simulink model "TCS_SlipModelControl"  (R2023b)
settings: Solver=VariableStepAuto  StartTime=0.0  StopTime=10.0  RelTol=1e-3
libraries: autolibim x1
settings Model: Creator=ibaad  LastModifiedBy=ibaad

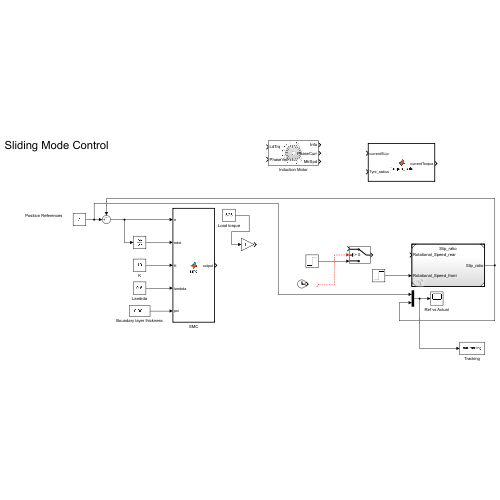
[thumbnail: Simulink's stored preview of the top-level diagram]
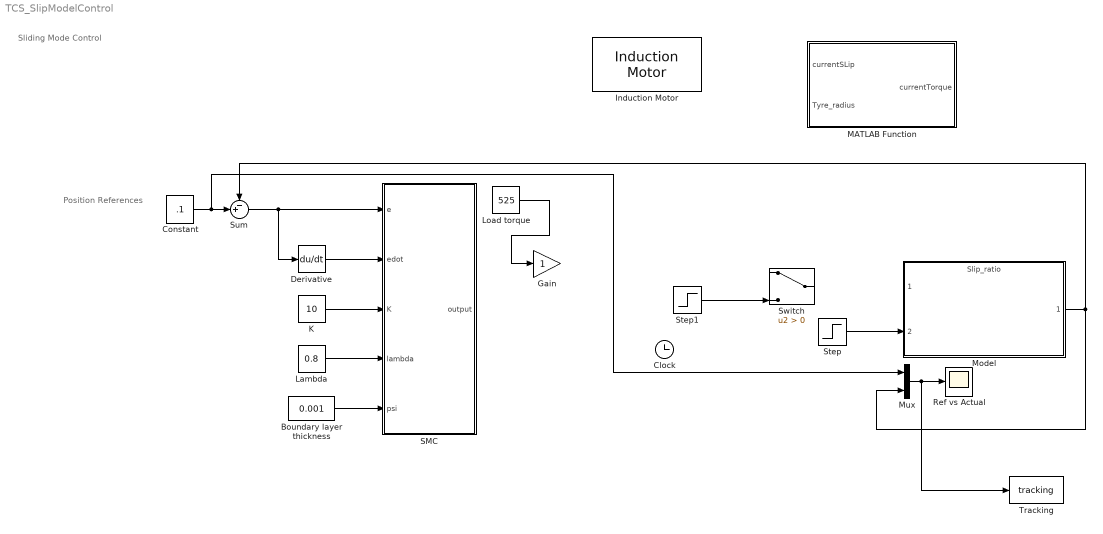
== system TCS_SlipModelControl ==
  note: Position References
  note: Sliding Mode Control
  Boundary layer thickness : Constant  Value=0.001
  Clock : Clock
  Constant : Constant  Value=.1
  Derivative : Derivative
  Gain : Gain
  Induction Motor : autolibim/Induction Motor  sim_type=Continuous  Ts=0.001  port_config=Torque  P=2  Zs=[1.77 0.0139]  Zr="[1.34  0.0121]"  Lm=0.3687  mechanical=[0.001 0 0]  theta_init=0  omega_init=0  RefBlkName='autolibim/Induction Motor'  aMode=5
      settings: LibrarySourceBlock=mcblib/Electrical Systems/Motors/Induction Motor
  K : Constant  Value=10
  Lambda : Constant  Value=0.8
  Load torque : Constant  Value=525
  MATLAB Function : MATLAB Function  TreatAsAtomicUnit=on
  Model : ModelReference  ModelNameDialog=Slip_ratio.slx  SimulationMode=Normal  ModelReferenceVersion=1.5
  Mux : Mux  Inputs=2
  Ref vs Actual : Scope
  SMC : MATLAB Function  TreatAsAtomicUnit=on
  Step : Step  Time=3  After=175  SampleTime=0
  Step1 : Step  SampleTime=0
  Sum : Sum  Inputs=-+|
  Switch : Switch  Criteria=u2 > Threshold  SaturateOnIntegerOverflow=off  InputSameDT=off
  Tracking : ToWorkspace  VariableName=tracking  SampleTime=-1
  wires:
  Sum/1 -> SMC/1(e), Derivative/1
  Derivative/1 -> SMC/2(edot)
  Boundary layer thickness/1 -> SMC/5(psi)
  Mux/1 -> Tracking/1, Ref vs Actual/1
  Lambda/1 -> SMC/4(lambda)
  K/1 -> SMC/3(K)
  Constant/1 -> Mux/1, Sum/2
  Model/1 -> Sum/1, Mux/2
  Step/1 -> Model/2
  Load torque/1 -> Gain/1
  Step1/1 -> Switch/3
  ? -> Switch/2

== matlab function TCS_SlipModelControl/MATLAB Function ==
  data: currentTorque output; currentSLip input; Tyre_radius input
function currentTorque = Torque_calc(currentSLip, Tyre_radius)
    % TCS_ACTIVE Summary of this function goes here

    e = exp(1); % Mathematical constant e
    % Friction curve as a function of slip ratio
    c1 = 1.2801; % Coef for dry asphalt
    c2 = 23.99; % Coef for dry asphalt
    c3 = 0.52; % Coef for dry asphalt
    Fn = 1350; % Normal force on one tire
    

 %   plot(slip_ratios, fricCoef); % Plot the entire array
 %   xlabel("Slip Ratio");
 %   ylabel("Longitudinal Friction Coefficient");
 %   title("Friction Coefficient vs. Slip Ratio Curve");
 %   grid on;% Optionally, turn the grid on for better readability


    fricCoef = c1 * (1 - exp(-c2 * currentSLip)) - c3 * currentSLip;
    currentTorque = ((fricCoef * Fn) * Tyre_radius);
end

== matlab function TCS_SlipModelControl/SMC ==
  data: e input; output output; edot input; K input; lambda input; psi input
function output = smc(e, edot, K, lambda, psi)
%#codegen

    s = lambda * e + edot;
        
    if (abs(s) > psi)    
        sat_s = sign(s);
    else
        sat_s = s/psi;
    end
    
    output = -(edot - K * sat_s);

end
